simulink model "Motor_Simulation_HBridge_doneLabor"  (R2018a)
settings: Solver=ode45  StartTime=0.0  StopTime=7.0  FixedStep=100e-6  RelTol=1e-3  EnableMultiTasking=on
values from neighbouring files (symbols this model uses):
  Cr = 7.2352*10^-6    (= 7.2352e-06)    [lab04_part01.m]    (also in lab05_part01_baga.m; lab06_simulationWithMeasurements.m)
  J = 5.5e-6    (= 5.5e-06)    [lab03_part01.m]    (also in lab04_part01.m = 8e-06; lab05_part01_baga.m = 8e-06; lab06_simulationWithMeasurements.m = 5.29e-06)
  ke = 0.017    [lab04_part01.m]    (also in lab05_part01_baga.m)
  km = 0.05    [lab04_part01.m]    (also in lab05_part01_baga.m)
  L = tan(phi).*Rges./(frequencies.*2*pi)    [lab02_part01.m]    (also in lab03_part01.m = 0.0005752; lab04_part01.m = 0.00035329; lab05_part01_baga.m = 0.00035329; lab06_simulationWithMeasurements.m = 0.000618)
  ML = 0    [lab04_part01.m]    (also in lab05_part01_baga.m)
  R = 3.71    [lab04_part01.m]
  Rshunt = 1    [lab04_part01.m]
settings Model: Creator=oleksandra  LastModifiedBy=oleksandra
settings DataIOCC: LimitDataPoints=on  SaveFormat=Array  SignalLoggingSaveFormat=ModelDataLogs
settings OptimizationCC: BlockReduction=off  BooleanDataType=off
settings DebuggingCC: SaveWithParameterizedLinksMsg=none  UnderspecifiedInitializationDetection=Classic  MergeDetectMultiDrivingBlocksExec=none  SignalResolutionControl=TryResolveAllWithWarning  MultiTaskDSMMsg=warning  MultiTaskCondExecSysMsg=none
settings HardwareCC: TargetUnknown=on
settings ModelReferenceCC: PropagateSignalLabelsOutOfModel=off
settings GRTTargetCC: TargetLangStandard=C89/C90 (ANSI)  CombineOutputUpdateFcns=off  GRTInterface=on
settings ConfigComp: CovHtmlReporting=on  CovSaveCumulativeToWorkspaceVar=on  CovSaveSingleToWorkspaceVar=on  CovExternalEMLEnable=off

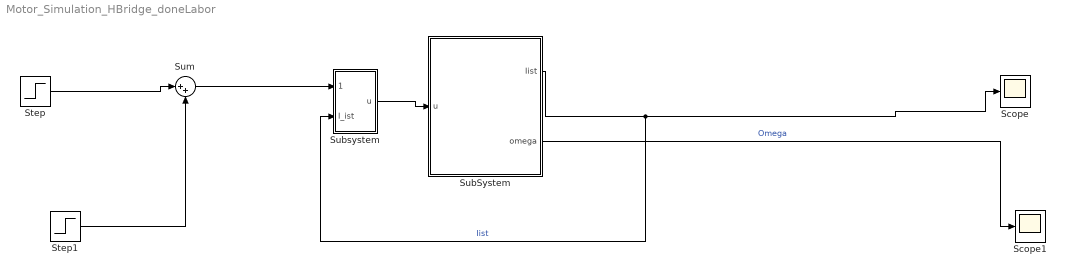
== system Motor_Simulation_HBridge_doneLabor ==
  Scope : Scope
  Scope1 : Scope
  Step : Step  Before=0.5  After=-0.3  SampleTime=0
  Step1 : Step  Time=4  After=0.9  SampleTime=0
  SubSystem : Subsystem
  Subsystem : Subsystem
  Sum : Sum  Inputs=|++  SaturateOnIntegerOverflow=on  InputSameDT=on  OutDataTypeStr=Inherit: Same as first input
  wires:
  SubSystem/1(Iist) -> Scope/1, Subsystem/2(I_ist)  "Iist"
  SubSystem/2(omega) -> Scope1/1  "Omega"
  Subsystem/1(u) -> SubSystem/1(u)
  Step/1 -> Sum/1
  Sum/1 -> Subsystem/1(I_soll)
  Step1/1 -> Sum/2

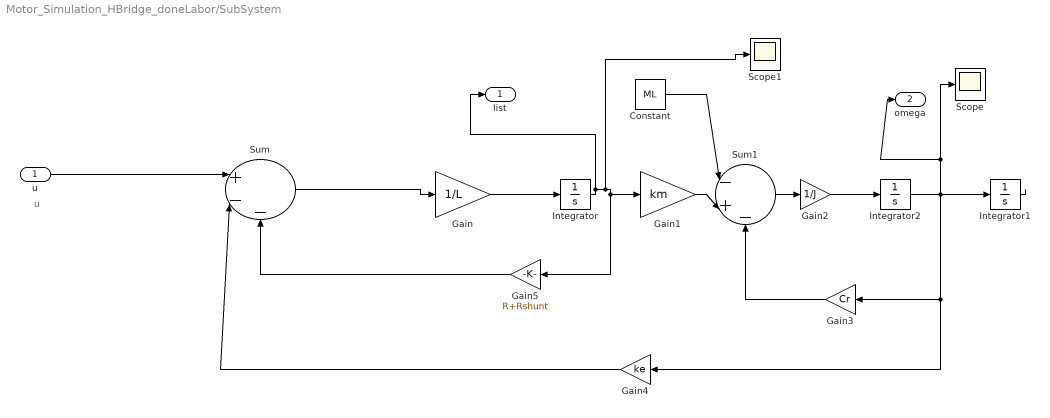
== system Motor_Simulation_HBridge_doneLabor/SubSystem ==
  note: u
  u : Inport  Description=output
  Constant : Constant  Value=ML
  Gain : Gain  Gain=1/L  SaturateOnIntegerOverflow=on  OutDataTypeStr=Inherit: Same as input  ParamDataTypeStr=Inherit: Same as input
  Gain1 : Gain  Gain=km  SaturateOnIntegerOverflow=on  OutDataTypeStr=Inherit: Same as input  ParamDataTypeStr=Inherit: Same as input
  Gain2 : Gain  Gain=1/J  SaturateOnIntegerOverflow=on  OutDataTypeStr=Inherit: Same as input  ParamDataTypeStr=Inherit: Same as input
  Gain3 : Gain  Gain=Cr  SaturateOnIntegerOverflow=on  OutDataTypeStr=Inherit: Same as input  ParamDataTypeStr=Inherit: Same as input
  Gain4 : Gain  Gain=ke  SaturateOnIntegerOverflow=on  OutDataTypeStr=Inherit: Same as input  ParamDataTypeStr=Inherit: Same as input
  Gain5 : Gain  Gain=R+Rshunt  SaturateOnIntegerOverflow=on  OutDataTypeStr=Inherit: Same as input  ParamDataTypeStr=Inherit: Same as input
  Integrator : Integrator
  Integrator1 : Integrator
  Integrator2 : Integrator
  Scope : Scope
  Scope1 : Scope
  Sum : Sum  Inputs=|+--  SaturateOnIntegerOverflow=on  InputSameDT=on  OutDataTypeStr=Inherit: Same as first input
  Sum1 : Sum  Inputs=|-+-  SaturateOnIntegerOverflow=on  InputSameDT=on  OutDataTypeStr=Inherit: Same as first input
  Iist : Outport
  omega : Outport  Port=2
  wires:
  Gain/1 -> Integrator/1
  Integrator/1 -> Iist/1, Gain1/1, Gain5/1, Scope1/1
  Sum/1 -> Gain/1
  Sum1/1 -> Gain2/1
  Gain2/1 -> Integrator2/1
  Integrator2/1 -> Scope/1, omega/1, Integrator1/1, Gain3/1, Gain4/1
  Gain4/1 -> Sum/2
  Gain3/1 -> Sum1/3
  Gain1/1 -> Sum1/2
  Gain5/1 -> Sum/3
  Constant/1 -> Sum1/1
  Integrator1/1 -> ?
  u/1 -> Sum/1

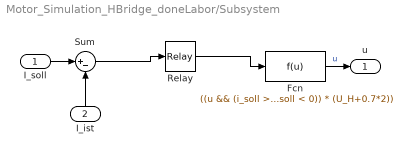
== system Motor_Simulation_HBridge_doneLabor/Subsystem ==
  I_soll : Inport
  I_ist : Inport  Port=2
  Fcn : Fcn  Expr=((u && (i_soll >= 0)) * (U_H)) + ((!u && (i_soll >= 0)) * (-U_H-0.7*2)) + ((!u && (i_soll < 0)) * (-U_H)) + ((u && (i_soll < 0)) * (U_H+0.7*2))
  Relay : Relay  OnSwitchValue=0.01  OffSwitchValue=-0.01
  Sum : Sum  Inputs=|+-  SaturateOnIntegerOverflow=on  InputSameDT=on  OutDataTypeStr=Inherit: Same as first input
  u : Outport
  wires:
  Relay/1 -> Fcn/1
  Sum/1 -> Relay/1
  I_soll/1 -> Sum/1
  Fcn/1 -> u/1  "u"
  I_ist/1 -> Sum/2
